simulink model "SUT_Test"  (Simulink 7.0)
settings: Solver=ode4  SolverMode=SingleTasking  StartTime=0.0  StopTime=252  FixedStep=0.01  RelTol=1e-3
InitFcn:
  | tempomat_para
StopFcn:
  | clear;
values from neighbouring files (symbols this model uses):
  A = 1.9    [tempomat_para.m]
  a_Fzg_max = 2    [tempomat_para.m]
  a_Fzg_min = -2    [tempomat_para.m]
  cw = 0.32    [tempomat_para.m]
  gang = [1 2 3 4]    [tempomat_para.m]
  gang_vec = [1 2 3 4]    [tempomat_para.m]
  i_anteil = 5    [tempomat_para.m]
  i_d = 3.42    [tempomat_para.m]
  i_g = [3.91 2.17 1.37 1.00]    [tempomat_para.m]
  lambda_gang = [1.3 1.25  1.17  1.05]    [tempomat_para.m]
  m_Fzg = 1400    [tempomat_para.m]
  M_mot_max = [130 149 163 170 168 166 162 158 150 139 123 80]    [tempomat_para.m]
  M_mot_min = [0 -40]    [tempomat_para.m]
  n_mot0 = 1000    [tempomat_para.m]
  n_mot_max = 1000:500:6500    [tempomat_para.m]
  n_mot_min = [1000 6500]    [tempomat_para.m]
  p_anteil = 100    [tempomat_para.m]
  r_dyn = 0.28    [tempomat_para.m]
  rho = 1.202    [tempomat_para.m]
  t_sch = 0.2    [tempomat_para.m]
  TI = [block '/TI']    [PSTI_callback.m]
  v_Fzg_ms0 = 0    [tempomat_para.m]
undefined symbols (not defined in the file or in its folder): Drossel_mat, getdatatypespecs
libraries: simulink x116, fzgbib x6
(part 2 of 11)

== system SUT_Test/Test Specification/R2 Speed Control velocity restoration time after simple  acceleration/deceleration/CC active + no target & Speed Control active & step of V_Des = |1|  with time periods >= 7s ==
  InOut Bus : Inport  OutDataType=sfix(16)  OutScaling=2^0
  Active : Constant  Value=2  OutDataType=sfix(16)  OutScaling=2^0
  Active + no target : Constant  Value=2  OutDataType=sfix(16)  OutScaling=2^0
  Bus Selector : BusSelector  OutputSignals=Inputs.signal3,Inputs.signal1,Inputs.signal2
  CC active & no target : Subsystem  mask(Range - Gap Absolute Tolerance){GorR=Range, AbsoluteTolerance=0}
      mask prompts: GorR "Use range or gap"; AbsoluteTolerance "Absolute Tolerance"
      mask help: Check that a signal stays inside a range or outside a gap around a reference signal. Specify the range or the gap absolute to the reference signal.
      mask init:
      | if max(get_param(gcb,'GorR') == ' ') % Gap
      |     helpVariable1 = '~=';
      | else % Range
      |     helpVariable1 = '==';
      | end
      | set_param([gcb '/Relational Operator'],'Operator',helpVariable1);
      mask StyleString: popup(Range|Gap  ),edit
      mask Display:
      | port_label('output',1,'A');
      | port_label('input',1,'Sig');
      | port_label('input',2,'Ref');
      | text(0.40,0.53,'+');
      | text(0.415,0.46,'-');
      | text(0.5,0.5,num2str(AbsoluteTolerance));
      | text(0.05,0.5,helpVariable1);
  CC active & no target1 : Subsystem  mask(Range - Gap Absolute Tolerance){GorR=Range, AbsoluteTolerance=0}
      mask prompts: GorR "Use range or gap"; AbsoluteTolerance "Absolute Tolerance"
      mask help: Check that a signal stays inside a range or outside a gap around a reference signal. Specify the range or the gap absolute to the reference signal.
      mask init:
      | if max(get_param(gcb,'GorR') == ' ') % Gap
      |     helpVariable1 = '~=';
      | else % Range
      |     helpVariable1 = '==';
      | end
      | set_param([gcb '/Relational Operator'],'Operator',helpVariable1);
      mask StyleString: popup(Range|Gap  ),edit
      mask Display:
      | port_label('output',1,'A');
      | port_label('input',1,'Sig');
      | port_label('input',2,'Ref');
      | text(0.40,0.53,'+');
      | text(0.415,0.46,'-');
      | text(0.5,0.5,num2str(AbsoluteTolerance));
      | text(0.05,0.5,helpVariable1);
  PS : Subsystem  mask(Feature layer: preconditions synchronization){NoTI=3, NoTDD=0, NoTID=0, TIdel=[0  0  0], TDDdel=[]}
      mask prompts: NoTI "Time-independent features identifiable with or without a delay (TI)"; NoTDD "Triggered features identifiable with determinate delay or without a delay (TDD)"; NoTID "Triggered features identifiable with indeterminate delay (TID)"; TIdel "Time-independent features delays (in time steps). E.g. [0 1 0] for 3 features"; TDDdel "Triggered features delays (in time steps). E.g. [0 0] for 2 features"
      mask help: Use this block for synchronizing the precondition features. For changing the block inputs, use the parameters below. The output must be used for assertions activation.
      mask init:
      | PS_init(gcb);
      mask StyleString: popup(0|1|2|3|4|5|6|7|8|9),popup(0|1|2|3|4|5|6|7|8|9),popup(0|1|2|3|4|5|6|7|8|9),edit,edit
      mask CallbackString:
      | PSTI_callback(gcb);|PSTDD_callback(gcb);|PSTID_callback(gcb);|NoTI = str2double(get_param(gcb,'NoTI'));
      | TIdel = str2num(get_param(gcb,'TIdel'));
      | if NoTI ~= length(TIdel) && NoTI ~= 0
      |     error(['The number of delays entered (' num2str(length(TIdel)) ') does not correspond to the above specified number of time-independent features (' num2str(NoTI) ').']);
      | end|NoTDD = str2double(get_param(gcb,'NoTDD'));
      | TDDdel = str2num(get_param(gcb,'TDDdel'));
      | if NoTDD ~= length(TDDdel) && NoTDD ~= 0
      |     error(['The number of delays entered (' num2str(length(TDDdel)) ') does not correspond to the above specified number of triggered features with constant delay (' num2str(NoTDD) ').']);
      | end
  Scope1 : Scope  NumInputPorts=3
      settings: TimeRange=120  YMin=-0.003370786516853574~-5~-5  YMax=0.3966292134831465~5~5  SaveName=ScopeData5  MaxDataPoints=5000000
  Speed Control active : Subsystem  mask(Range - Gap Absolute Tolerance){GorR=Range, AbsoluteTolerance=0}
      mask prompts: GorR "Use range or gap"; AbsoluteTolerance "Absolute Tolerance"
      mask help: Check that a signal stays inside a range or outside a gap around a reference signal. Specify the range or the gap absolute to the reference signal.
      mask init:
      | if max(get_param(gcb,'GorR') == ' ') % Gap
      |     helpVariable1 = '~=';
      | else % Range
      |     helpVariable1 = '==';
      | end
      | set_param([gcb '/Relational Operator'],'Operator',helpVariable1);
      mask StyleString: popup(Range|Gap  ),edit
      mask Display:
      | port_label('output',1,'A');
      | port_label('input',1,'Sig');
      | port_label('input',2,'Ref');
      | text(0.40,0.53,'+');
      | text(0.415,0.46,'-');
      | text(0.5,0.5,num2str(AbsoluteTolerance));
      | text(0.05,0.5,helpVariable1);
  Step with step size=|1|  and time periods >= 6s detection : Subsystem  mask(Complete step detection){Param=0}
      mask prompts: Param "Mask Parameter 1:"
  true : Constant  OutDataType=sfix(16)  OutScaling=2^0
  Activate : Outport  OutDataType=sfix(16)  OutScaling=2^0
  wires:
  PS/1(Precond) -> Activate/1
  InOut Bus/1 -> Bus Selector/1
  Bus Selector/1 -> Step with step size=|1|  and time periods >= 6s detection/1(Step)  "<signal3>"
  Bus Selector/2 -> CC active & no target/1(Signal)  "<signal1>"
  Active + no target/1 -> CC active & no target/2(Reference)
  Active/1 -> Speed Control active/2(Reference)
  Bus Selector/3 -> Speed Control active/1(Signal)  "<signal2>"
  Step with step size=|1|  and time periods >= 6s detection/1(Complete step) -> CC active & no target1/1(Signal)
  true/1 -> CC active & no target1/2(Reference)
  CC active & no target1/1(Activate) -> PS/1(A TI1)
  CC active & no target/1(Activate) -> PS/2(A TI2)
  Speed Control active/1(Activate) -> PS/3(A TI3)

== system SUT_Test/Test Specification/R2 Speed Control velocity restoration time after simple  acceleration/deceleration/after (6 seconds)  |V_Des-V_Vhcl <= 1.4| ==
  Precond : Inport  OutDataType=sfix(16)  OutScaling=2^0
  InOut Bus : Inport  Port=2  OutDataType=sfix(16)  OutScaling=2^0
  " " : Subsystem  mask(Bound){cm=<=, Lower=1, Upper=0, Ass=[1 2], Pre=[1 2], Req=[1 2]}
      mask prompts: cm "Comparison method:"; Upper "Mask Parameter 3:"; Req "Mask Parameter 6:"
      mask help:
      | Compare a signal with a reference using the specified comparison method.
      |
      | Output verdict V and lower (LL) and upper (UL) limits for reporting.
      |
      | For '==' or '~=' use "Range - Gap"
      mask init: same as SUT_Test/Test Specification/R1 Speed Control step response/Maximum overshoot < 5 &  Steady state error < 5/Maximum overshoot < 5
      mask StyleString: popup(>|>=|<=|<),edit,edit,edit,edit,edit
      mask Display:
      | port_label('output', 1, ['V']);
      | port_label('input', 1, 'Sig');
      | port_label('input', 2, 'Ref');
      | text(0.05,0.5,get_param(get_param([get_param(gcb,'Parent') '/' get_param(gcb,'Name') '/Relational Operator'],'handle'),'Operator'));
  Bus Creator : BusCreator  Inputs=1
  Bus Selector : BusSelector  OutputSignals=Inputs.signal3,Outputs.signal1
  Bus Selector{1..4} (4 alike) : BusSelector  OutputSignals=Local verdict
  PAS1 : Subsystem  mask{AFT=TI, AFD=600}
      mask prompts: AFT "Assertion feature type:"; AFD "Assertion feature delay (in time steps)"
      mask init:
      | PAS_init(gcb);
      mask StyleString: popup(TI|TDD|TID),edit
      mask CallbackString: PAS_callback(gcb);|
  PAS2 : Subsystem  mask{AFT=TI, AFD=600}
      mask prompts: AFT "Assertion feature type:"; AFD "Assertion feature delay (in time steps)"
      mask init:
      | PAS_init(gcb);
      mask StyleString: popup(TI|TDD|TID),edit
      mask CallbackString: PAS_callback(gcb);|
  R = 2 : Subsystem
  Scope : Scope  NumInputPorts=5
      settings: YMin=-5~-5~-5~80~0  YMax=5~5~5~107.5~110  SaveName=ScopeData2  MaxDataPoints=5000000
  t1 : Constant  Value=1.4  OutDataType=sfix(16)  OutScaling=2^0
  t2 : Constant  OutDataType=sfix(16)  OutScaling=2^0
  within(20 sec)1 : Subsystem  mask(Bound){cm=<=, Lower=1, Upper=0, Ass=[1 2], Pre=[1 2], Req=[1 2]}
      mask prompts: cm "Comparison method:"; Upper "Mask Parameter 3:"; Req "Mask Parameter 6:"
      mask help:
      | Compare a signal with a reference using the specified comparison method.
      |
      | Output verdict V and lower (LL) and upper (UL) limits for reporting.
      |
      | For '==' or '~=' use "Range - Gap"
      mask init: same as SUT_Test/Test Specification/R1 Speed Control step response/Maximum overshoot < 5 &  Steady state error < 5/Maximum overshoot < 5
      mask StyleString: popup(>|>=|<=|<),edit,edit,edit,edit,edit
      mask Display:
      | port_label('output', 1, ['V']);
      | port_label('input', 1, 'Sig');
      | port_label('input', 2, 'Ref');
      | text(0.05,0.5,get_param(get_param([get_param(gcb,'Parent') '/' get_param(gcb,'Name') '/Relational Operator'],'handle'),'Operator'));
  |V_Des-V_Vhcl| : Subsystem
  VF info : Outport  OutDataType=sfix(16)  OutScaling=2^0
  wires:
  t1/1 -> " "/2(Reference)
  " "/1(V) -> Bus Selector1/1, PAS1/2(V)
  InOut Bus/1 -> |V_Des-V_Vhcl|/1(InOut Bus), Bus Selector/1, R = 2/2(In2)
  Bus Creator/1 -> VF info/1
  Precond/1 -> PAS1/1(Precond), PAS2/1(Precond), R = 2/1(In1)
  PAS1/1(VF Info) -> Bus Creator/1, Bus Selector2/1
  |V_Des-V_Vhcl|/1(Out1) -> " "/1(Signal)
  t2/1 -> within(20 sec)1/2(Reference)
  within(20 sec)1/1(V) -> Bus Selector4/1, PAS2/2(V)
  R = 2/1(Out1) -> within(20 sec)1/1(Signal), Scope/3
  Bus Selector4/1 -> Scope/1  "<Local verdict>"
  PAS2/1(VF Info) -> Bus Selector3/1
  Bus Selector3/1 -> Scope/2  "<Local verdict>"

== system SUT_Test/SUT/ Speed Controller /Compute SUC inputs/Oneway-Filter ==
  note: 21.5.1997/Hoetzer/FKFS
  in : Inport  OutDataType=sfix(16)  OutScaling=2^0
  1/T : Fcn  Expr=1/u
  Fcn : Fcn  Expr=u[1]<-0.01
  Fcn1 : Fcn  Expr=u[1]<0.01
  Grenze3 : Constant  Value=zk  OutDataType=sfix(16)  OutScaling=2^0
  Grenze4 : Constant  Value=0.1  OutDataType=sfix(16)  OutScaling=2^0
  Integrator : Integrator
  Logical Operator : Logic  Operator=OR
  Logical Operator1 : Logic
  Product : Product  OutDataType=sfix(16)  OutScaling=2^0  SaturateOnIntegerOverflow=on  InputSameDT=on
  Reglerabweichung : Sum  Inputs=-+  OutDataType=sfix(16)  OutScaling=2^0  SaturateOnIntegerOverflow=on  InputSameDT=on
  Relational Operator1 : RelationalOperator  InputSameDT=on
  Switch : Switch  Threshold=0.5  SaturateOnIntegerOverflow=on  InputSameDT=on
  reale Ableitung : TransferFcn  Numerator=[1 0]  Denominator=[0.1 1]
  "out " : Outport  OutDataType=sfix(16)  OutScaling=2^0  InitialOutput=0
  wires:
  Relational Operator1/1 -> Logical Operator1/2
  Fcn/1 -> Logical Operator1/1
  reale Ableitung/1 -> Fcn/1
  Grenze3/1 -> Switch/3
  Grenze4/1 -> Switch/1
  in/1 -> Relational Operator1/2, Fcn1/1, reale Ableitung/1, Reglerabweichung/2
  1/T/1 -> Product/2
  Reglerabweichung/1 -> Product/1
  Switch/1 -> 1/T/1
  Logical Operator/1 -> Switch/2
  Product/1 -> Integrator/1
  Integrator/1 -> Relational Operator1/1, Reglerabweichung/1, "out "/1
  Fcn1/1 -> Logical Operator/2
  Logical Operator1/1 -> Logical Operator/1

== system SUT_Test/SUT/ Speed Controller /Compute SUC inputs/neg_Beschleunigungsbegrenzung ==
  note: Das Bremsmoment wird solange durchgereicht, solange die Beschleunigung > -2 ist.
      | Im anderen Fall wird das in diesem Fall gespeicherte Bremsmoment durchgereicht.
  M_Br_v : Inport  OutDataType=sfix(16)  OutScaling=2^0
  a_Fzg_mss : Inport  Port=2  OutDataType=sfix(16)  OutScaling=2^0
  M_Br_n : Inport  Port=3  OutDataType=sfix(16)  OutScaling=2^0
  Constant1 : Constant  Value=a_Fzg_min  OutDataType=sfix(16)  OutScaling=2^0
  Data Store Memory : DataStoreMemory  DataStoreName=M_Br2  OutDataType=sfix(16)  OutScaling=2^0
  Data Store Read : DataStoreRead  DataStoreName=M_Br2  SampleTime=-1
  Gangspeicher : Memory  X0=1
  Logical Operator : Logic  Operator=OR
  Logical Operator1 : Logic  Orientation=down  Operator=NOT  Inputs=1
  Relational Operator : RelationalOperator  Operator=>  InputSameDT=on
  Relational Operator1 : RelationalOperator  Operator=<=  InputSameDT=on
  Reset M_Br2 : Subsystem  TreatAsAtomicUnit=on
  Switch : Switch  Threshold=0.5  SaturateOnIntegerOverflow=on  InputSameDT=on
  tw5 : ToWorkspace  VariableName=b_l  SaveFormat=Array
      settings: MaxDataPoints=speicher
  tw6 : ToWorkspace  VariableName=M_Br2  SaveFormat=Array
      settings: MaxDataPoints=speicher
  tw7 : ToWorkspace  VariableName=M_Br1  SaveFormat=Array
      settings: MaxDataPoints=speicher
  M_Br3 : Outport  OutDataType=sfix(16)  OutScaling=2^0  InitialOutput=0
  wires:
  Switch/1 -> M_Br3/1
  Constant1/1 -> Relational Operator/2
  Relational Operator1/1 -> Logical Operator/2
  Data Store Read/1 -> Switch/3, tw6/1, Relational Operator1/2
  Logical Operator/1 -> Gangspeicher/1
  Gangspeicher/1 -> Switch/2, tw5/1
  M_Br_n/1 -> Reset M_Br2/1(M_Br_n)
  M_Br_v/1 -> Switch/1, tw7/1, Relational Operator1/1
  Relational Operator/1 -> Logical Operator/1, Logical Operator1/1
  Logical Operator1/1 -> Reset M_Br2/Enable
  a_Fzg_mss/1 -> Relational Operator/1, Reset M_Br2/2(a_Fzg_mss)

== system SUT_Test/SUT/ Speed Controller /Compute SUC inputs/pos_Beschleunigungsbegrenzung ==
  note: Das Bremsmoment wird solange durchgereicht, solange die Beschleunigung > -2 ist.
      | Im anderen Fall wird das in diesem Fall gespeicherte Bremsmoment durchgereicht.
  M_Mot_v : Inport  OutDataType=sfix(16)  OutScaling=2^0
  a_Fzg_mss : Inport  Port=2  OutDataType=sfix(16)  OutScaling=2^0
  "n_Mot " : Inport  Port=3  OutDataType=sfix(16)  OutScaling=2^0
  Constant1 : Constant  Value=a_Fzg_max  OutDataType=sfix(16)  OutScaling=2^0
  Data Store Memory : DataStoreMemory  DataStoreName=M_Mot2  OutDataType=sfix(16)  OutScaling=2^0
  Data Store Read : DataStoreRead  DataStoreName=M_Mot2  SampleTime=-1
  Gangspeicher : Memory  X0=1
  Logical Operator : Logic  Operator=OR
  Logical Operator1 : Logic  Orientation=down  Operator=NOT  Inputs=1
  MinMax : MinMax  Inputs=2  OutDataType=sfix(16)  OutScaling=2^0  SaturateOnIntegerOverflow=on  InputSameDT=on
  Relational Operator : RelationalOperator  Operator=<  InputSameDT=on
  Relational Operator1 : RelationalOperator  Operator=<=  InputSameDT=on
  Reset M_Mot2 : Subsystem  TreatAsAtomicUnit=on
  Switch : Switch  Threshold=0.5  SaturateOnIntegerOverflow=on  InputSameDT=on
  maximales Motormoment : Lookup  InputValues=[0 n_mot_max]  Table=[M_mot_max(1) M_mot_max]  OutDataType=sfix(16)  OutScaling=2^0  SaturateOnIntegerOverflow=on
  tw5 : ToWorkspace  VariableName=b_l2  SaveFormat=Array
      settings: MaxDataPoints=speicher
  tw6 : ToWorkspace  VariableName=M_Mot2  SaveFormat=Array
      settings: MaxDataPoints=speicher
  tw7 : ToWorkspace  VariableName=M_Mot1  SaveFormat=Array
      settings: MaxDataPoints=speicher
  M_Mot3 : Outport  OutDataType=sfix(16)  OutScaling=2^0  InitialOutput=0
  wires:
  Switch/1 -> M_Mot3/1
  Constant1/1 -> Relational Operator/2
  Relational Operator1/1 -> Logical Operator/2
  Data Store Read/1 -> Switch/3, tw6/1, Relational Operator1/2
  Logical Operator/1 -> Gangspeicher/1
  Gangspeicher/1 -> Switch/2, tw5/1
  M_Mot_v/1 -> Switch/1, tw7/1, Relational Operator1/1, MinMax/1
  Relational Operator/1 -> Logical Operator/1, Logical Operator1/1
  Logical Operator1/1 -> Reset M_Mot2/Enable
  a_Fzg_mss/1 -> Relational Operator/1
  MinMax/1 -> Reset M_Mot2/1(M_Mot_n)
  "n_Mot "/1 -> maximales Motormoment/1
  maximales Motormoment/1 -> MinMax/2

== system SUT_Test/SUT/ Speed Controller /Speed Controller/Regler ==
  d_v : Inport  OutDataType=sfix(16)  OutScaling=2^0
  Integrator : Integrator  LimitOutput=on  UpperSaturationLimit=2000  LowerSaturationLimit=-2000
  P_Anteil : Gain  Gain=p_anteil  ParameterDataType=sfix(16)  ParameterScaling=2^0  OutDataType=sfix(16)  OutScaling=2^0  SaturateOnIntegerOverflow=on
  Sum : Sum  OutDataType=sfix(16)  OutScaling=2^0  SaturateOnIntegerOverflow=on  InputSameDT=on
  "m/s -> km/h1" : Gain  Gain=i_anteil  ParameterDataType=sfix(16)  ParameterScaling=2^0  OutDataType=sfix(16)  OutScaling=2^0  SaturateOnIntegerOverflow=on
  "u_R " : Outport  OutDataType=sfix(16)  OutScaling=2^0  InitialOutput=0
  wires:
  Sum/1 -> "u_R "/1
  P_Anteil/1 -> Sum/1
  "m/s -> km/h1"/1 -> Integrator/1
  d_v/1 -> P_Anteil/1, "m/s -> km/h1"/1
  Integrator/1 -> Sum/2

== system SUT_Test/SUT/ Speed Controller /Speed Controller/Stoergroessenkompensation ==
  v_Fzg : Inport  OutDataType=sfix(16)  OutScaling=2^0
  v_soll : Inport  Port=2  OutDataType=sfix(16)  OutScaling=2^0
  GR_aktiv_l : Inport  Port=3  OutDataType=sfix(16)  OutScaling=2^0
  Luft- und Rollwiderstand : Subsystem
  P-Anteil : Gain  Gain=3000  ParameterDataType=sfix(16)  ParameterScaling=2^0  OutDataType=sfix(16)  OutScaling=2^0  SaturateOnIntegerOverflow=on
  P-Anteil1 : Gain  Gain=m_Fzg  ParameterDataType=sfix(16)  ParameterScaling=2^0  OutDataType=sfix(16)  OutScaling=2^0  SaturateOnIntegerOverflow=on
  Sollverhalten Fahrzeug mit P-Regler1 : Subsystem
  Sum : Sum  Inputs=2  OutDataType=sfix(16)  OutScaling=2^0  SaturateOnIntegerOverflow=on  InputSameDT=on
  Sum1 : Sum  Inputs=2  OutDataType=sfix(16)  OutScaling=2^0  SaturateOnIntegerOverflow=on  InputSameDT=on
  Sum2 : Sum  Inputs=+-  OutDataType=sfix(16)  OutScaling=2^0  SaturateOnIntegerOverflow=on  InputSameDT=on
  r_dyn : Gain  Gain=r_dyn  ParameterDataType=sfix(16)  ParameterScaling=2^0  OutDataType=sfix(16)  OutScaling=2^0  SaturateOnIntegerOverflow=on
  reale Ableitung : TransferFcn  Numerator=[1 0]  Denominator=[0.5 1]
  u_s : Outport  OutDataType=sfix(16)  OutScaling=2^0  InitialOutput=0
  wires:
  Sum1/1 -> Sum/2
  Luft- und Rollwiderstand/1(M_G) -> Sum/1
  P-Anteil/1 -> Sum1/2
  P-Anteil1/1 -> Sum1/1
  Sollverhalten Fahrzeug mit P-Regler1/1(v_Fzg1) -> Sum2/1
  r_dyn/1 -> P-Anteil1/1
  GR_aktiv_l/1 -> Sollverhalten Fahrzeug mit P-Regler1/3(GR_aktiv_l)
  reale Ableitung/1 -> r_dyn/1
  v_soll/1 -> Sollverhalten Fahrzeug mit P-Regler1/1(v_soll)
  Sum2/1 -> reale Ableitung/1, P-Anteil/1
  v_Fzg/1 -> Sollverhalten Fahrzeug mit P-Regler1/2(v_Fzg), Sum2/2, Luft- und Rollwiderstand/1(v_Fzg)
  Sum/1 -> u_s/1

== system SUT_Test/SUT/Vehicle Model/Fahrzeugmodell/Drosselklappenstellung ==
  n_mot : Inport  OutDataType=sfix(16)  OutScaling=2^0
  M_Mot_b : Inport  Port=2  OutDataType=sfix(16)  OutScaling=2^0
  schalt_l : Inport  Port=3  OutDataType=sfix(16)  OutScaling=2^0
  Constant : Constant  Value=0  OutDataType=sfix(16)  OutScaling=2^0
  Constant1 : Constant  Value=n_mot0+100  OutDataType=sfix(16)  OutScaling=2^0
  Constant2 : Constant  Value=0  OutDataType=sfix(16)  OutScaling=2^0
  Drosselklappenkennfeld : Lookup2D  RowIndex=n_Mot_vec  ColumnIndex=M_Mot_vec  Table=Drossel_mat  OutDataType=sfix(16)  OutScaling=2^0  SaturateOnIntegerOverflow=on  InputSameDT=on
  Logical Operator : Logic
  Logical Operator1 : Logic  Operator=OR
  PT1 Filterung : TransferFcn  Denominator=[0.1 1]
  Relational Operator : RelationalOperator  InputSameDT=on
  Relational Operator1 : RelationalOperator  Operator=<=  InputSameDT=on
  Saturation : Saturate  UpperLimit=90  LowerLimit=0
  Switch : Switch  Threshold=0.5  SaturateOnIntegerOverflow=on  InputSameDT=on
  damit bei Vollast 90 Grad : Fcn  Expr=u+3
  DK_Stellung [Grad] : Outport  OutDataType=sfix(16)  OutScaling=2^0  InitialOutput=0
  wires:
  Relational Operator1/1 -> Logical Operator/2
  Relational Operator/1 -> Logical Operator/1
  Logical Operator/1 -> Logical Operator1/1
  schalt_l/1 -> Logical Operator1/2
  Constant/1 -> Switch/1
  Logical Operator1/1 -> Switch/2
  Constant2/1 -> Relational Operator1/2
  Constant1/1 -> Relational Operator/2
  Saturation/1 -> PT1 Filterung/1
  PT1 Filterung/1 -> DK_Stellung [Grad]/1
  Switch/1 -> Saturation/1
  M_Mot_b/1 -> Relational Operator1/1, Drosselklappenkennfeld/2
  n_mot/1 -> Relational Operator/1, Drosselklappenkennfeld/1
  Drosselklappenkennfeld/1 -> damit bei Vollast 90 Grad/1
  damit bei Vollast 90 Grad/1 -> Switch/3

== system SUT_Test/SUT/Vehicle Model/Fahrzeugmodell/Fahrwiderstaende ==
  note: Widerstandskraefte
  note: Keine Steigung beruecksichtigt
  M_Mot_b : Inport  OutDataType=sfix(16)  OutScaling=2^0
  M_Br_b : Inport  Port=2  OutDataType=sfix(16)  OutScaling=2^0
  Gang_w : Inport  Port=3  OutDataType=sfix(16)  OutScaling=2^0
  v_Fzg_ms : Inport  Port=4  OutDataType=sfix(16)  OutScaling=2^0
  F_A Berechnung ausgekuppelt : Constant  Value=0  OutDataType=sfix(16)  OutScaling=2^0
  F_A Berechnung eingekuppelt : Fcn  Expr=u[1]*u[2]*i_d/r_dyn
  F_Brems Berechnung : Fcn  Expr=(u[1]>0)*u[2]/r_dyn
  F_L Berechnung : Fcn  Expr=u*rho*A/2*cw
  F_R Berechnung : Fcn  Expr=(u>0.1)*f_r*m_Fzg*g
  Gesamtgetriebe- uebersetzung : Fcn  Expr=u*i_d
  Getriebeuebersetzung : Lookup  InputValues=gang  Table=i_g  OutDataType=sfix(16)  OutScaling=2^0  SaturateOnIntegerOverflow=on
  Mux : Mux  Inputs=2
  Mux1 : Mux  Inputs=2
  Product : Product  OutDataType=sfix(16)  OutScaling=2^0  SaturateOnIntegerOverflow=on  InputSameDT=on
  Schaltdauer : Subsystem
  Switch : Switch  Threshold=0.5  SaturateOnIntegerOverflow=on  InputSameDT=on
  Zeit bis Gang  eingelegt ist : TransportDelay  DelayTime=t_sch  InitialOutput=1
  tw3 : ToWorkspace  VariableName=k_l  SaveFormat=Array
      settings: MaxDataPoints=speicher
  F_A : Outport  OutDataType=sfix(16)  OutScaling=2^0  InitialOutput=0
  F_L : Outport  Port=2  OutDataType=sfix(16)  OutScaling=2^0  InitialOutput=0
  F_R : Outport  Port=3  OutDataType=sfix(16)  OutScaling=2^0  InitialOutput=0
  F_Brems : Outport  Port=4  OutDataType=sfix(16)  OutScaling=2^0  InitialOutput=0
  i_gesamt : Outport  Port=5  OutDataType=sfix(16)  OutScaling=2^0  InitialOutput=0
  Gang_i : Outport  Port=6  OutDataType=sfix(16)  OutScaling=2^0  InitialOutput=0
  schalt_l : Outport  Port=7  OutDataType=sfix(16)  OutScaling=2^0  InitialOutput=0
  wires:
  F_L Berechnung/1 -> F_L/1
  Product/1 -> F_L Berechnung/1
  v_Fzg_ms/1 -> Product/2, Product/1, F_R Berechnung/1, Mux1/1
  F_Brems Berechnung/1 -> F_Brems/1
  F_R Berechnung/1 -> F_R/1
  Mux1/1 -> F_Brems Berechnung/1
  M_Br_b/1 -> Mux1/2
  Schaltdauer/1(k_l) -> schalt_l/1, Switch/2, tw3/1
  F_A Berechnung eingekuppelt/1 -> Switch/3
  M_Mot_b/1 -> Mux/2
  Mux/1 -> F_A Berechnung eingekuppelt/1
  Gesamtgetriebe- uebersetzung/1 -> i_gesamt/1
  Getriebeuebersetzung/1 -> Mux/1, Gesamtgetriebe- uebersetzung/1
  Switch/1 -> F_A/1
  Gang_w/1 -> Getriebeuebersetzung/1, Schaltdauer/1(Gang_w), Zeit bis Gang  eingelegt ist/1
  F_A Berechnung ausgekuppelt/1 -> Switch/1
  Zeit bis Gang  eingelegt ist/1 -> Gang_i/1

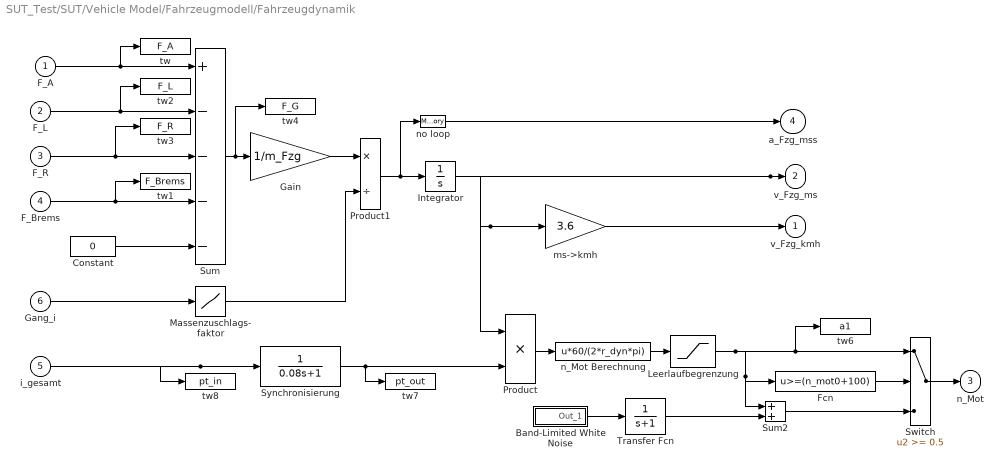
== system SUT_Test/SUT/Vehicle Model/Fahrzeugmodell/Fahrzeugdynamik ==
  F_A : Inport  OutDataType=sfix(16)  OutScaling=2^0
  F_L : Inport  Port=2  OutDataType=sfix(16)  OutScaling=2^0
  F_R : Inport  Port=3  OutDataType=sfix(16)  OutScaling=2^0
  F_Brems : Inport  Port=4  OutDataType=sfix(16)  OutScaling=2^0
  i_gesamt : Inport  Port=5  OutDataType=sfix(16)  OutScaling=2^0
  Gang_i : Inport  Port=6  OutDataType=sfix(16)  OutScaling=2^0
  Band-Limited White Noise : Subsystem  mask(Continuous White Noise.){@1=[3], @2=0.2, @3=[23341]}
      mask prompts: @1 "Noise Power:"; @2 "Sample Time:"; @3 "Seed"
      mask help:
      | White noise for continuous (s-domain) systems.
      | Band-limited using zero-order-hold.
      mask init:
      | Cov = @1; Ts = @2; seed = @3; r = rand(1,12); r2 = [r(1),r;r,r(12)]; t =[1:13;1:13];
      mask Help: Implemented using white noise into Zero-Order Hold block. The seed and power can be vectors of the same length to produce a vector of white noise sources. For faster simulation, set sample time to the highest value possible but in accordance with the fastest dynamics of system.
      mask Display: plot(t(:),r2(:))
  Constant : Constant  Value=0  OutDataType=sfix(16)  OutScaling=2^0
  Fcn : Fcn  Expr=u>=(n_mot0+100)
  Gain : Gain  Gain=1/m_Fzg  ParameterDataType=sfix(16)  ParameterScaling=2^0  OutDataType=sfix(16)  OutScaling=2^0  SaturateOnIntegerOverflow=on
  Integrator : Integrator  InitialCondition=v_Fzg_ms0  UpperSaturationLimit=100  LowerSaturationLimit=0
  Leerlaufbegrenzung : Saturate  UpperLimit=7000  LowerLimit=n_mot0
  Massenzuschlags- faktor : Lookup  InputValues=gang_vec  Table=lambda_gang  OutDataType=sfix(16)  OutScaling=2^0  SaturateOnIntegerOverflow=on
  Product : Product  OutDataType=sfix(16)  OutScaling=2^0  SaturateOnIntegerOverflow=on  InputSameDT=on
  Product1 : Product  Inputs=*/  OutDataType=sfix(16)  OutScaling=2^0  SaturateOnIntegerOverflow=on  InputSameDT=on
  Sum : Sum  Inputs=+----  OutDataType=sfix(16)  OutScaling=2^0  SaturateOnIntegerOverflow=on  InputSameDT=on
  Sum2 : Sum  OutDataType=sfix(16)  OutScaling=2^0  SaturateOnIntegerOverflow=on  InputSameDT=on
  Switch : Switch  Threshold=0.5  SaturateOnIntegerOverflow=on  InputSameDT=on
  Synchronisierung : TransferFcn  Denominator=[0.08 1]
  Transfer Fcn : TransferFcn  Denominator=[1 1]
  ms->kmh : Gain  Gain=3.6  ParameterDataType=sfix(16)  ParameterScaling=2^0  OutDataType=sfix(16)  OutScaling=2^0  SaturateOnIntegerOverflow=on
  n_Mot Berechnung : Fcn  Expr=u*60/(2*r_dyn*pi)
  no loop : Memory
  tw : ToWorkspace  VariableName=F_A  SaveFormat=Array
      settings: MaxDataPoints=speicher
  tw1 : ToWorkspace  VariableName=F_Brems  SaveFormat=Array
      settings: MaxDataPoints=speicher
  tw2 : ToWorkspace  VariableName=F_L  SaveFormat=Array
      settings: MaxDataPoints=speicher
  tw3 : ToWorkspace  VariableName=F_R  SaveFormat=Array
      settings: MaxDataPoints=speicher
  tw4 : ToWorkspace  VariableName=F_G  SaveFormat=Array
      settings: MaxDataPoints=speicher
  tw6 : ToWorkspace  VariableName=a1  SaveFormat=Array
      settings: MaxDataPoints=speicher
  tw7 : ToWorkspace  VariableName=pt_out  SaveFormat=Array
      settings: MaxDataPoints=speicher
  tw8 : ToWorkspace  VariableName=pt_in  SaveFormat=Array
      settings: MaxDataPoints=speicher
  v_Fzg_kmh : Outport  OutDataType=sfix(16)  OutScaling=2^0  InitialOutput=0
  v_Fzg_ms : Outport  Port=2  OutDataType=sfix(16)  OutScaling=2^0  InitialOutput=0
  n_Mot : Outport  Port=3  OutDataType=sfix(16)  OutScaling=2^0  InitialOutput=0
  a_Fzg_mss : Outport  Port=4  OutDataType=sfix(16)  OutScaling=2^0  InitialOutput=0
  wires:
  Constant/1 -> Sum/5
  F_Brems/1 -> tw1/1, Sum/4
  F_R/1 -> Sum/3, tw3/1
  F_L/1 -> Sum/2, tw2/1
  F_A/1 -> tw/1, Sum/1
  ms->kmh/1 -> v_Fzg_kmh/1
  Integrator/1 -> Product/1, ms->kmh/1, v_Fzg_ms/1
  no loop/1 -> a_Fzg_mss/1
  Product/1 -> n_Mot Berechnung/1
  n_Mot Berechnung/1 -> Leerlaufbegrenzung/1
  Gang_i/1 -> Massenzuschlags- faktor/1
  Massenzuschlags- faktor/1 -> Product1/2
  Product1/1 -> no loop/1, Integrator/1
  Gain/1 -> Product1/1
  Sum/1 -> Gain/1, tw4/1
  Synchronisierung/1 -> Product/2, tw7/1
  i_gesamt/1 -> Synchronisierung/1, tw8/1
  Fcn/1 -> Switch/2
  Sum2/1 -> Switch/3
  Leerlaufbegrenzung/1 -> tw6/1, Switch/1, Sum2/1, Fcn/1
  Transfer Fcn/1 -> Sum2/2
  Band-Limited White Noise/1(Out_1) -> Transfer Fcn/1
  Switch/1 -> n_Mot/1

== system SUT_Test/SUT / Speed Controller /Compute SUC inputs/Oneway-Filter ==
  note: 21.5.1997/Hoetzer/FKFS
  in : Inport  OutDataType=sfix(16)  OutScaling=2^0
  1/T : Fcn  Expr=1/u
  Fcn : Fcn  Expr=u[1]<-0.01
  Fcn1 : Fcn  Expr=u[1]<0.01
  Grenze3 : Constant  Value=zk  OutDataType=sfix(16)  OutScaling=2^0
  Grenze4 : Constant  Value=0.1  OutDataType=sfix(16)  OutScaling=2^0
  Integrator : Integrator
  Logical Operator : Logic  Operator=OR
  Logical Operator1 : Logic
  Product : Product  OutDataType=sfix(16)  OutScaling=2^0  SaturateOnIntegerOverflow=on  InputSameDT=on
  Reglerabweichung : Sum  Inputs=-+  OutDataType=sfix(16)  OutScaling=2^0  SaturateOnIntegerOverflow=on  InputSameDT=on
  Relational Operator1 : RelationalOperator  InputSameDT=on
  Switch : Switch  Threshold=0.5  SaturateOnIntegerOverflow=on  InputSameDT=on
  reale Ableitung : TransferFcn  Numerator=[1 0]  Denominator=[0.1 1]
  "out " : Outport  OutDataType=sfix(16)  OutScaling=2^0  InitialOutput=0
  wires:
  Relational Operator1/1 -> Logical Operator1/2
  Fcn/1 -> Logical Operator1/1
  reale Ableitung/1 -> Fcn/1
  Grenze3/1 -> Switch/3
  Grenze4/1 -> Switch/1
  in/1 -> Relational Operator1/2, Fcn1/1, reale Ableitung/1, Reglerabweichung/2
  1/T/1 -> Product/2
  Reglerabweichung/1 -> Product/1
  Switch/1 -> 1/T/1
  Logical Operator/1 -> Switch/2
  Product/1 -> Integrator/1
  Integrator/1 -> Relational Operator1/1, Reglerabweichung/1, "out "/1
  Fcn1/1 -> Logical Operator/2
  Logical Operator1/1 -> Logical Operator/1

== system SUT_Test/SUT / Speed Controller /Compute SUC inputs/neg_Beschleunigungsbegrenzung ==
  note: Das Bremsmoment wird solange durchgereicht, solange die Beschleunigung > -2 ist.
      | Im anderen Fall wird das in diesem Fall gespeicherte Bremsmoment durchgereicht.
  M_Br_v : Inport  OutDataType=sfix(16)  OutScaling=2^0
  a_Fzg_mss : Inport  Port=2  OutDataType=sfix(16)  OutScaling=2^0
  M_Br_n : Inport  Port=3  OutDataType=sfix(16)  OutScaling=2^0
  Constant1 : Constant  Value=a_Fzg_min  OutDataType=sfix(16)  OutScaling=2^0
  Data Store Memory : DataStoreMemory  DataStoreName=M_Br2  OutDataType=sfix(16)  OutScaling=2^0
  Data Store Read : DataStoreRead  DataStoreName=M_Br2  SampleTime=-1
  Gangspeicher : Memory  X0=1
  Logical Operator : Logic  Operator=OR
  Logical Operator1 : Logic  Orientation=down  Operator=NOT  Inputs=1
  Relational Operator : RelationalOperator  Operator=>  InputSameDT=on
  Relational Operator1 : RelationalOperator  Operator=<=  InputSameDT=on
  Reset M_Br2 : Subsystem  TreatAsAtomicUnit=on
  Switch : Switch  Threshold=0.5  SaturateOnIntegerOverflow=on  InputSameDT=on
  tw5 : ToWorkspace  VariableName=b_l  SaveFormat=Array
      settings: MaxDataPoints=speicher
  tw6 : ToWorkspace  VariableName=M_Br2  SaveFormat=Array
      settings: MaxDataPoints=speicher
  tw7 : ToWorkspace  VariableName=M_Br1  SaveFormat=Array
      settings: MaxDataPoints=speicher
  M_Br3 : Outport  OutDataType=sfix(16)  OutScaling=2^0  InitialOutput=0
  wires:
  Switch/1 -> M_Br3/1
  Constant1/1 -> Relational Operator/2
  Relational Operator1/1 -> Logical Operator/2
  Data Store Read/1 -> Switch/3, tw6/1, Relational Operator1/2
  Logical Operator/1 -> Gangspeicher/1
  Gangspeicher/1 -> Switch/2, tw5/1
  M_Br_n/1 -> Reset M_Br2/1(M_Br_n)
  M_Br_v/1 -> Switch/1, tw7/1, Relational Operator1/1
  Relational Operator/1 -> Logical Operator/1, Logical Operator1/1
  Logical Operator1/1 -> Reset M_Br2/Enable
  a_Fzg_mss/1 -> Relational Operator/1, Reset M_Br2/2(a_Fzg_mss)

== system SUT_Test/SUT / Speed Controller /Compute SUC inputs/pos_Beschleunigungsbegrenzung ==
  note: Das Bremsmoment wird solange durchgereicht, solange die Beschleunigung > -2 ist.
      | Im anderen Fall wird das in diesem Fall gespeicherte Bremsmoment durchgereicht.
  M_Mot_v : Inport  OutDataType=sfix(16)  OutScaling=2^0
  a_Fzg_mss : Inport  Port=2  OutDataType=sfix(16)  OutScaling=2^0
  "n_Mot " : Inport  Port=3  OutDataType=sfix(16)  OutScaling=2^0
  Constant1 : Constant  Value=a_Fzg_max  OutDataType=sfix(16)  OutScaling=2^0
  Data Store Memory : DataStoreMemory  DataStoreName=M_Mot2  OutDataType=sfix(16)  OutScaling=2^0
  Data Store Read : DataStoreRead  DataStoreName=M_Mot2  SampleTime=-1
  Gangspeicher : Memory  X0=1
  Logical Operator : Logic  Operator=OR
  Logical Operator1 : Logic  Orientation=down  Operator=NOT  Inputs=1
  MinMax : MinMax  Inputs=2  OutDataType=sfix(16)  OutScaling=2^0  SaturateOnIntegerOverflow=on  InputSameDT=on
  Relational Operator : RelationalOperator  Operator=<  InputSameDT=on
  Relational Operator1 : RelationalOperator  Operator=<=  InputSameDT=on
  Reset M_Mot2 : Subsystem  TreatAsAtomicUnit=on
  Switch : Switch  Threshold=0.5  SaturateOnIntegerOverflow=on  InputSameDT=on
  maximales Motormoment : Lookup  InputValues=[0 n_mot_max]  Table=[M_mot_max(1) M_mot_max]  OutDataType=sfix(16)  OutScaling=2^0  SaturateOnIntegerOverflow=on
  tw5 : ToWorkspace  VariableName=b_l2  SaveFormat=Array
      settings: MaxDataPoints=speicher
  tw6 : ToWorkspace  VariableName=M_Mot2  SaveFormat=Array
      settings: MaxDataPoints=speicher
  tw7 : ToWorkspace  VariableName=M_Mot1  SaveFormat=Array
      settings: MaxDataPoints=speicher
  M_Mot3 : Outport  OutDataType=sfix(16)  OutScaling=2^0  InitialOutput=0
  wires:
  Switch/1 -> M_Mot3/1
  Constant1/1 -> Relational Operator/2
  Relational Operator1/1 -> Logical Operator/2
  Data Store Read/1 -> Switch/3, tw6/1, Relational Operator1/2
  Logical Operator/1 -> Gangspeicher/1
  Gangspeicher/1 -> Switch/2, tw5/1
  M_Mot_v/1 -> Switch/1, tw7/1, Relational Operator1/1, MinMax/1
  Relational Operator/1 -> Logical Operator/1, Logical Operator1/1
  Logical Operator1/1 -> Reset M_Mot2/Enable
  a_Fzg_mss/1 -> Relational Operator/1
  MinMax/1 -> Reset M_Mot2/1(M_Mot_n)
  "n_Mot "/1 -> maximales Motormoment/1
  maximales Motormoment/1 -> MinMax/2

== system SUT_Test/SUT / Speed Controller /Speed Controller/Regler ==
  d_v : Inport  OutDataType=sfix(16)  OutScaling=2^0
  Integrator : Integrator  LimitOutput=on  UpperSaturationLimit=2000  LowerSaturationLimit=-2000
  P_Anteil : Gain  Gain=p_anteil  ParameterDataType=sfix(16)  ParameterScaling=2^0  OutDataType=sfix(16)  OutScaling=2^0  SaturateOnIntegerOverflow=on
  Sum : Sum  OutDataType=sfix(16)  OutScaling=2^0  SaturateOnIntegerOverflow=on  InputSameDT=on
  "m/s -> km/h1" : Gain  Gain=i_anteil  ParameterDataType=sfix(16)  ParameterScaling=2^0  OutDataType=sfix(16)  OutScaling=2^0  SaturateOnIntegerOverflow=on
  "u_R " : Outport  OutDataType=sfix(16)  OutScaling=2^0  InitialOutput=0
  wires:
  Sum/1 -> "u_R "/1
  P_Anteil/1 -> Sum/1
  "m/s -> km/h1"/1 -> Integrator/1
  d_v/1 -> P_Anteil/1, "m/s -> km/h1"/1
  Integrator/1 -> Sum/2

== system SUT_Test/SUT / Speed Controller /Speed Controller/Stoergroessenkompensation ==
  v_Fzg : Inport  OutDataType=sfix(16)  OutScaling=2^0
  v_soll : Inport  Port=2  OutDataType=sfix(16)  OutScaling=2^0
  GR_aktiv_l : Inport  Port=3  OutDataType=sfix(16)  OutScaling=2^0
  Luft- und Rollwiderstand : Subsystem
  P-Anteil : Gain  Gain=3000  ParameterDataType=sfix(16)  ParameterScaling=2^0  OutDataType=sfix(16)  OutScaling=2^0  SaturateOnIntegerOverflow=on
  P-Anteil1 : Gain  Gain=m_Fzg  ParameterDataType=sfix(16)  ParameterScaling=2^0  OutDataType=sfix(16)  OutScaling=2^0  SaturateOnIntegerOverflow=on
  Sollverhalten Fahrzeug mit P-Regler1 : Subsystem
  Sum : Sum  Inputs=2  OutDataType=sfix(16)  OutScaling=2^0  SaturateOnIntegerOverflow=on  InputSameDT=on
  Sum1 : Sum  Inputs=2  OutDataType=sfix(16)  OutScaling=2^0  SaturateOnIntegerOverflow=on  InputSameDT=on
  Sum2 : Sum  Inputs=+-  OutDataType=sfix(16)  OutScaling=2^0  SaturateOnIntegerOverflow=on  InputSameDT=on
  r_dyn : Gain  Gain=r_dyn  ParameterDataType=sfix(16)  ParameterScaling=2^0  OutDataType=sfix(16)  OutScaling=2^0  SaturateOnIntegerOverflow=on
  reale Ableitung : TransferFcn  Numerator=[1 0]  Denominator=[0.5 1]
  u_s : Outport  OutDataType=sfix(16)  OutScaling=2^0  InitialOutput=0
  wires:
  Sum1/1 -> Sum/2
  Luft- und Rollwiderstand/1(M_G) -> Sum/1
  P-Anteil/1 -> Sum1/2
  P-Anteil1/1 -> Sum1/1
  Sollverhalten Fahrzeug mit P-Regler1/1(v_Fzg1) -> Sum2/1
  r_dyn/1 -> P-Anteil1/1
  GR_aktiv_l/1 -> Sollverhalten Fahrzeug mit P-Regler1/3(GR_aktiv_l)
  reale Ableitung/1 -> r_dyn/1
  v_soll/1 -> Sollverhalten Fahrzeug mit P-Regler1/1(v_soll)
  Sum2/1 -> reale Ableitung/1, P-Anteil/1
  v_Fzg/1 -> Sollverhalten Fahrzeug mit P-Regler1/2(v_Fzg), Sum2/2, Luft- und Rollwiderstand/1(v_Fzg)
  Sum/1 -> u_s/1

== system SUT_Test/SUT /Vehicle Model/Fahrzeugmodell/Drosselklappenstellung ==
  n_mot : Inport  OutDataType=sfix(16)  OutScaling=2^0
  M_Mot_b : Inport  Port=2  OutDataType=sfix(16)  OutScaling=2^0
  schalt_l : Inport  Port=3  OutDataType=sfix(16)  OutScaling=2^0
  Constant : Constant  Value=0  OutDataType=sfix(16)  OutScaling=2^0
  Constant1 : Constant  Value=n_mot0+100  OutDataType=sfix(16)  OutScaling=2^0
  Constant2 : Constant  Value=0  OutDataType=sfix(16)  OutScaling=2^0
  Drosselklappenkennfeld : Lookup2D  RowIndex=n_Mot_vec  ColumnIndex=M_Mot_vec  Table=Drossel_mat  OutDataType=sfix(16)  OutScaling=2^0  SaturateOnIntegerOverflow=on  InputSameDT=on
  Logical Operator : Logic
  Logical Operator1 : Logic  Operator=OR
  PT1 Filterung : TransferFcn  Denominator=[0.1 1]
  Relational Operator : RelationalOperator  InputSameDT=on
  Relational Operator1 : RelationalOperator  Operator=<=  InputSameDT=on
  Saturation : Saturate  UpperLimit=90  LowerLimit=0
  Switch : Switch  Threshold=0.5  SaturateOnIntegerOverflow=on  InputSameDT=on
  damit bei Vollast 90 Grad : Fcn  Expr=u+3
  DK_Stellung [Grad] : Outport  OutDataType=sfix(16)  OutScaling=2^0  InitialOutput=0
  wires:
  Relational Operator1/1 -> Logical Operator/2
  Relational Operator/1 -> Logical Operator/1
  Logical Operator/1 -> Logical Operator1/1
  schalt_l/1 -> Logical Operator1/2
  Constant/1 -> Switch/1
  Logical Operator1/1 -> Switch/2
  Constant2/1 -> Relational Operator1/2
  Constant1/1 -> Relational Operator/2
  Saturation/1 -> PT1 Filterung/1
  PT1 Filterung/1 -> DK_Stellung [Grad]/1
  Switch/1 -> Saturation/1
  M_Mot_b/1 -> Relational Operator1/1, Drosselklappenkennfeld/2
  n_mot/1 -> Relational Operator/1, Drosselklappenkennfeld/1
  Drosselklappenkennfeld/1 -> damit bei Vollast 90 Grad/1
  damit bei Vollast 90 Grad/1 -> Switch/3

== system SUT_Test/SUT /Vehicle Model/Fahrzeugmodell/Fahrwiderstaende ==
  note: Widerstandskraefte
  note: Keine Steigung beruecksichtigt
  M_Mot_b : Inport  OutDataType=sfix(16)  OutScaling=2^0
  M_Br_b : Inport  Port=2  OutDataType=sfix(16)  OutScaling=2^0
  Gang_w : Inport  Port=3  OutDataType=sfix(16)  OutScaling=2^0
  v_Fzg_ms : Inport  Port=4  OutDataType=sfix(16)  OutScaling=2^0
  F_A Berechnung ausgekuppelt : Constant  Value=0  OutDataType=sfix(16)  OutScaling=2^0
  F_A Berechnung eingekuppelt : Fcn  Expr=u[1]*u[2]*i_d/r_dyn
  F_Brems Berechnung : Fcn  Expr=(u[1]>0)*u[2]/r_dyn
  F_L Berechnung : Fcn  Expr=u*rho*A/2*cw
  F_R Berechnung : Fcn  Expr=(u>0.1)*f_r*m_Fzg*g
  Gesamtgetriebe- uebersetzung : Fcn  Expr=u*i_d
  Getriebeuebersetzung : Lookup  InputValues=gang  Table=i_g  OutDataType=sfix(16)  OutScaling=2^0  SaturateOnIntegerOverflow=on
  Mux : Mux  Inputs=2
  Mux1 : Mux  Inputs=2
  Product : Product  OutDataType=sfix(16)  OutScaling=2^0  SaturateOnIntegerOverflow=on  InputSameDT=on
  Schaltdauer : Subsystem
  Switch : Switch  Threshold=0.5  SaturateOnIntegerOverflow=on  InputSameDT=on
  Zeit bis Gang  eingelegt ist : TransportDelay  DelayTime=t_sch  InitialOutput=1
  tw3 : ToWorkspace  VariableName=k_l  SaveFormat=Array
      settings: MaxDataPoints=speicher
  F_A : Outport  OutDataType=sfix(16)  OutScaling=2^0  InitialOutput=0
  F_L : Outport  Port=2  OutDataType=sfix(16)  OutScaling=2^0  InitialOutput=0
  F_R : Outport  Port=3  OutDataType=sfix(16)  OutScaling=2^0  InitialOutput=0
  F_Brems : Outport  Port=4  OutDataType=sfix(16)  OutScaling=2^0  InitialOutput=0
  i_gesamt : Outport  Port=5  OutDataType=sfix(16)  OutScaling=2^0  InitialOutput=0
  Gang_i : Outport  Port=6  OutDataType=sfix(16)  OutScaling=2^0  InitialOutput=0
  schalt_l : Outport  Port=7  OutDataType=sfix(16)  OutScaling=2^0  InitialOutput=0
  wires:
  F_L Berechnung/1 -> F_L/1
  Product/1 -> F_L Berechnung/1
  v_Fzg_ms/1 -> Product/2, Product/1, F_R Berechnung/1, Mux1/1
  F_Brems Berechnung/1 -> F_Brems/1
  F_R Berechnung/1 -> F_R/1
  Mux1/1 -> F_Brems Berechnung/1
  M_Br_b/1 -> Mux1/2
  Schaltdauer/1(k_l) -> schalt_l/1, Switch/2, tw3/1
  F_A Berechnung eingekuppelt/1 -> Switch/3
  M_Mot_b/1 -> Mux/2
  Mux/1 -> F_A Berechnung eingekuppelt/1
  Gesamtgetriebe- uebersetzung/1 -> i_gesamt/1
  Getriebeuebersetzung/1 -> Mux/1, Gesamtgetriebe- uebersetzung/1
  Switch/1 -> F_A/1
  Gang_w/1 -> Getriebeuebersetzung/1, Schaltdauer/1(Gang_w), Zeit bis Gang  eingelegt ist/1
  F_A Berechnung ausgekuppelt/1 -> Switch/1
  Zeit bis Gang  eingelegt ist/1 -> Gang_i/1

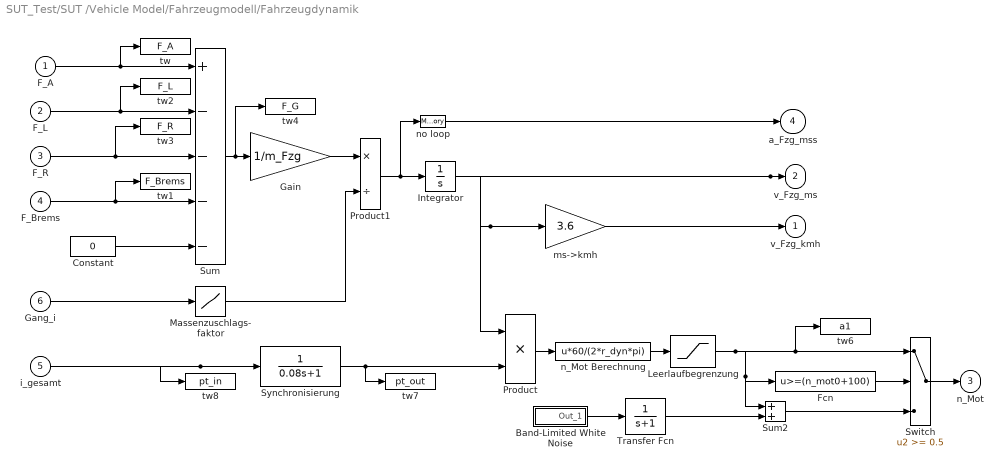
== system SUT_Test/SUT /Vehicle Model/Fahrzeugmodell/Fahrzeugdynamik ==
  F_A : Inport  OutDataType=sfix(16)  OutScaling=2^0
  F_L : Inport  Port=2  OutDataType=sfix(16)  OutScaling=2^0
  F_R : Inport  Port=3  OutDataType=sfix(16)  OutScaling=2^0
  F_Brems : Inport  Port=4  OutDataType=sfix(16)  OutScaling=2^0
  i_gesamt : Inport  Port=5  OutDataType=sfix(16)  OutScaling=2^0
  Gang_i : Inport  Port=6  OutDataType=sfix(16)  OutScaling=2^0
  Band-Limited White Noise : Subsystem  mask(Continuous White Noise.){@1=[3], @2=0.2, @3=[23341]}
      mask prompts: @1 "Noise Power:"; @2 "Sample Time:"; @3 "Seed"
      mask help:
      | White noise for continuous (s-domain) systems.
      | Band-limited using zero-order-hold.
      mask init:
      | Cov = @1; Ts = @2; seed = @3; r = rand(1,12); r2 = [r(1),r;r,r(12)]; t =[1:13;1:13];
      mask Help: Implemented using white noise into Zero-Order Hold block. The seed and power can be vectors of the same length to produce a vector of white noise sources. For faster simulation, set sample time to the highest value possible but in accordance with the fastest dynamics of system.
      mask Display: plot(t(:),r2(:))
  Constant : Constant  Value=0  OutDataType=sfix(16)  OutScaling=2^0
  Fcn : Fcn  Expr=u>=(n_mot0+100)
  Gain : Gain  Gain=1/m_Fzg  ParameterDataType=sfix(16)  ParameterScaling=2^0  OutDataType=sfix(16)  OutScaling=2^0  SaturateOnIntegerOverflow=on
  Integrator : Integrator  InitialCondition=v_Fzg_ms0  UpperSaturationLimit=100  LowerSaturationLimit=0
  Leerlaufbegrenzung : Saturate  UpperLimit=7000  LowerLimit=n_mot0
  Massenzuschlags- faktor : Lookup  InputValues=gang_vec  Table=lambda_gang  OutDataType=sfix(16)  OutScaling=2^0  SaturateOnIntegerOverflow=on
  Product : Product  OutDataType=sfix(16)  OutScaling=2^0  SaturateOnIntegerOverflow=on  InputSameDT=on
  Product1 : Product  Inputs=*/  OutDataType=sfix(16)  OutScaling=2^0  SaturateOnIntegerOverflow=on  InputSameDT=on
  Sum : Sum  Inputs=+----  OutDataType=sfix(16)  OutScaling=2^0  SaturateOnIntegerOverflow=on  InputSameDT=on
  Sum2 : Sum  OutDataType=sfix(16)  OutScaling=2^0  SaturateOnIntegerOverflow=on  InputSameDT=on
  Switch : Switch  Threshold=0.5  SaturateOnIntegerOverflow=on  InputSameDT=on
  Synchronisierung : TransferFcn  Denominator=[0.08 1]
  Transfer Fcn : TransferFcn  Denominator=[1 1]
  ms->kmh : Gain  Gain=3.6  ParameterDataType=sfix(16)  ParameterScaling=2^0  OutDataType=sfix(16)  OutScaling=2^0  SaturateOnIntegerOverflow=on
  n_Mot Berechnung : Fcn  Expr=u*60/(2*r_dyn*pi)
  no loop : Memory
  tw : ToWorkspace  VariableName=F_A  SaveFormat=Array
      settings: MaxDataPoints=speicher
  tw1 : ToWorkspace  VariableName=F_Brems  SaveFormat=Array
      settings: MaxDataPoints=speicher
  tw2 : ToWorkspace  VariableName=F_L  SaveFormat=Array
      settings: MaxDataPoints=speicher
  tw3 : ToWorkspace  VariableName=F_R  SaveFormat=Array
      settings: MaxDataPoints=speicher
  tw4 : ToWorkspace  VariableName=F_G  SaveFormat=Array
      settings: MaxDataPoints=speicher
  tw6 : ToWorkspace  VariableName=a1  SaveFormat=Array
      settings: MaxDataPoints=speicher
  tw7 : ToWorkspace  VariableName=pt_out  SaveFormat=Array
      settings: MaxDataPoints=speicher
  tw8 : ToWorkspace  VariableName=pt_in  SaveFormat=Array
      settings: MaxDataPoints=speicher
  v_Fzg_kmh : Outport  OutDataType=sfix(16)  OutScaling=2^0  InitialOutput=0
  v_Fzg_ms : Outport  Port=2  OutDataType=sfix(16)  OutScaling=2^0  InitialOutput=0
  n_Mot : Outport  Port=3  OutDataType=sfix(16)  OutScaling=2^0  InitialOutput=0
  a_Fzg_mss : Outport  Port=4  OutDataType=sfix(16)  OutScaling=2^0  InitialOutput=0
  wires:
  Constant/1 -> Sum/5
  F_Brems/1 -> tw1/1, Sum/4
  F_R/1 -> Sum/3, tw3/1
  F_L/1 -> Sum/2, tw2/1
  F_A/1 -> tw/1, Sum/1
  ms->kmh/1 -> v_Fzg_kmh/1
  Integrator/1 -> Product/1, ms->kmh/1, v_Fzg_ms/1
  no loop/1 -> a_Fzg_mss/1
  Product/1 -> n_Mot Berechnung/1
  n_Mot Berechnung/1 -> Leerlaufbegrenzung/1
  Gang_i/1 -> Massenzuschlags- faktor/1
  Massenzuschlags- faktor/1 -> Product1/2
  Product1/1 -> no loop/1, Integrator/1
  Gain/1 -> Product1/1
  Sum/1 -> Gain/1, tw4/1
  Synchronisierung/1 -> Product/2, tw7/1
  i_gesamt/1 -> Synchronisierung/1, tw8/1
  Fcn/1 -> Switch/2
  Sum2/1 -> Switch/3
  Leerlaufbegrenzung/1 -> tw6/1, Switch/1, Sum2/1, Fcn/1
  Transfer Fcn/1 -> Sum2/2
  Band-Limited White Noise/1(Out_1) -> Transfer Fcn/1
  Switch/1 -> n_Mot/1

== system SUT_Test/Test Data/R1 Speed Control step response/Complete step & CC active + no target & Speed Control active/Generate complete step ==
  Out Bus : Inport  OutDataType=sfix(16)  OutScaling=2^0
  " " : RelationalOperator  Operator===  LogicOutDataTypeMode=boolean
  Bus Selector : BusSelector  OutputSignals=signal2.signal1.signal1.signal2.T
  Clock1 : Clock
      settings: Decimation=10
  Data Store : DataStoreMemory  DataStoreName=triggerTime  OutDataType=sfix(16)  OutScaling=2^0
  Generate step : Step  InitFcn=triggerTime=150  Time=85.4+const  Before=XF  After=XF+size  SampleTime=0  VectorParams1D=off
  "Generate step " : Step  Time=t  Before=XO  After=XF  SampleTime=0
  Hold Time : Subsystem  TreatAsAtomicUnit=on
  Hold Value : Subsystem  TreatAsAtomicUnit=on
  Memory : Memory
  Switch : Switch  Criteria=u2 > Threshold
  triggered : Constant  OutDataType=sfix(16)  OutScaling=2^0
  v_Des : Outport  OutDataType=sfix(16)  OutScaling=2^0
  wires:
  Out Bus/1 -> Bus Selector/1
  triggered/1 -> " "/2
  " "/1 -> Hold Value/1(trigger), Hold Value/Enable, Hold Time/Enable
  Generate step/1 -> Switch/1
  "Generate step "/1 -> Switch/3
  Switch/1 -> v_Des/1
  Hold Value/1(triggered) -> Switch/2
  Clock1/1 -> Hold Time/1(Clock)
  Memory/1 -> " "/1
  Bus Selector/1 -> Memory/1  "<T>"

== system SUT_Test/Test Data/R2 Speed Control velocity restoration time after simple  acceleration/deceleration/ CC active + no target & Speed Control active & V_Des increases/decreases  7 times by 1 unit/V_Des increases/decreases  7 times by 1 unit ==
  Generate step : Step  InitFcn=triggerTime=150  Time=147+7  Before=50  After=51  SampleTime=0  VectorParams1D=off
  Generate step1 : Step  InitFcn=triggerTime=150  Time=147+7+42+7  After=-1  SampleTime=0  VectorParams1D=off
  Step : Step  Time=147+7+21  SampleTime=0
  Step1 : Step  Time=147+7+35  SampleTime=0
  Step10 : Step  Time=147+7+42+7+28  After=-1  SampleTime=0
  Step11 : Step  Time=147+7+42+7+42  After=-1  SampleTime=0
  Step2 : Step  Time=147+7+14  SampleTime=0
  Step3 : Step  Time=147+7+7  SampleTime=0
  Step4 : Step  Time=147+7+42+7+21  After=-1  SampleTime=0
  Step5 : Step  Time=147+7+28  SampleTime=0
  Step6 : Step  Time=147+7+42  SampleTime=0
  Step7 : Step  Time=147+7+42+7+35  After=-1  SampleTime=0
  Step8 : Step  Time=147+7+42+7+14  After=-2  SampleTime=0
  Step9 : Step  Time=147+7+42+7+7  After=-1  SampleTime=0
  Sum1 : Sum  Inputs=+++++++  OutDataType=sfix(16)  OutScaling=2^0
  Sum2 : Sum  Inputs=+++++++  OutDataType=sfix(16)  OutScaling=2^0
  Sum3 : Sum  OutDataType=sfix(16)  OutScaling=2^0
  v_Des : Outport  OutDataType=sfix(16)  OutScaling=2^0
  wires:
  Sum2/1 -> Sum3/1
  Sum1/1 -> Sum3/2
  Sum3/1 -> v_Des/1
  Generate step/1 -> Sum1/1
  Step3/1 -> Sum1/2
  Step2/1 -> Sum1/3
  Step/1 -> Sum1/4
  Step5/1 -> Sum1/5
  Step1/1 -> Sum1/6
  Step6/1 -> Sum1/7
  Generate step1/1 -> Sum2/1
  Step9/1 -> Sum2/2
  Step8/1 -> Sum2/3
  Step4/1 -> Sum2/4
  Step10/1 -> Sum2/5
  Step7/1 -> Sum2/6
  Step11/1 -> Sum2/7

== system SUT_Test/Test Specification/R1 Speed Control step response/Complete step & CC active + no target & Speed Control active/CC active & no target ==
  Signal : Inport  OutDataType=sfix(16)  OutScaling=2^0
  Reference : Inport  Port=2  OutDataType=sfix(16)  OutScaling=2^0
  Abs : Abs
  Abs1 : Abs
  Absolute Tolerance : Constant  Value=AbsoluteTolerance  OutDataType=sfix(16)  OutScaling=2^0
  Add : Sum  Inputs=+-  OutDataType=sfix(16)  OutScaling=2^-10
  Relational Operator : RelationalOperator  Operator===  LogicOutDataTypeMode=boolean
  Activate : Outport  OutDataType=sfix(16)  OutScaling=2^0
  wires:
  Relational Operator/1 -> Activate/1
  Abs/1 -> Relational Operator/1
  Add/1 -> Abs/1
  Signal/1 -> Add/1
  Reference/1 -> Add/2
  Absolute Tolerance/1 -> Abs1/1
  Abs1/1 -> Relational Operator/2
